simulink model "MASs"  (R2015b)
settings: Solver=ode45  SolverMode=SingleTasking  StartTime=0.0  StopTime=100000.0  RelTol=1e-3
model workspace (MAT data in the model file):
  B = 3.17
  Cb = 0.251
  Izz = 1
  L = 9.8
  d = 0.71
  m = 5540
undefined symbols (not defined in the file or in its folder): magnitude
libraries: simulink x10
(part 2 of 2)

== system MASs/usv3/USV/F model/S model ==
  u : Inport
  v : Inport  Port=2
  r : Inport  Port=3
  B : Constant  Value=B
  Cb : Constant  Value=Cb
  L : Constant  Value=L
  d : Constant  Value=d
  m : Constant  Value=m
  s-fcn : MATLAB Function  TreatAsAtomicUnit=on
  Xs : Outport
  Ys : Outport  Port=2
  Ns : Outport  Port=3
  wires:
  s-fcn/1(Xs) -> Xs/1
  s-fcn/2(Ys) -> Ys/1
  s-fcn/3(Ns) -> Ns/1
  B/1 -> s-fcn/1(B)
  d/1 -> s-fcn/2(d)
  L/1 -> s-fcn/3(L)
  u/1 -> s-fcn/6(u)
  v/1 -> s-fcn/7(v)
  r/1 -> s-fcn/8(r)
  Cb/1 -> s-fcn/4(Cb)
  m/1 -> s-fcn/5(m)

== system MASs/usv3/USV/F model/W model ==
  n : Constant  Value=0
  n1 : Constant  Value=0
  n2 : Constant  Value=0
  Xw : Outport
  Yw : Outport  Port=2
  Nw : Outport  Port=3
  wires:
  n/1 -> Xw/1
  n2/1 -> Yw/1
  n1/1 -> Nw/1

== system MASs/usv3/USV/motion model/r-sub ==
  N : Inport
  Izz : Inport  Port=2
  Jzz : Inport  Port=3
  Divide2 : Product  Inputs=*/
  Integrator2 : Integrator
  Sum4 : Sum  Inputs=|++
  r : Outport
  wires:
  Sum4/1 -> Divide2/2
  Divide2/1 -> Integrator2/1  "r'"
  Integrator2/1 -> r/1  "r"
  N/1 -> Divide2/1
  Jzz/1 -> Sum4/2
  Izz/1 -> Sum4/1

== system MASs/usv3/USV/motion model/u-sub ==
  X : Inport
  m : Inport  Port=2
  my : Inport  Port=3
  mx : Inport  Port=4
  v : Inport  Port=5
  r : Inport  Port=6
  Add : Sum
  Divide1 : Product  Inputs=*/
  Integrator : Integrator
  Product : Product  Inputs=3
  Sum : Sum  Inputs=|++
  Sum1 : Sum  Inputs=|++
  u : Outport
  wires:
  Sum1/1 -> Divide1/2
  Divide1/1 -> Integrator/1  "u'"
  Integrator/1 -> u/1  "u"
  Sum/1 -> Product/1
  Add/1 -> Divide1/1
  my/1 -> Sum/2
  X/1 -> Add/1
  v/1 -> Product/2
  r/1 -> Product/3
  mx/1 -> Sum1/2
  m/1 -> Sum1/1, Sum/1
  Product/1 -> Add/2

== system MASs/usv3/USV/motion model/v-sub ==
  Y : Inport
  m : Inport  Port=2
  mx : Inport  Port=3
  my : Inport  Port=4
  u : Inport  Port=5
  r : Inport  Port=6
  Add2 : Sum  Inputs=+-
  Divide3 : Product  Inputs=*/
  Integrator1 : Integrator
  Product1 : Product  Inputs=3
  Sum2 : Sum  Inputs=|++
  Sum3 : Sum  Inputs=|++
  v : Outport
  wires:
  Sum3/1 -> Divide3/2
  my/1 -> Sum3/1
  r/1 -> Product1/3
  Product1/1 -> Add2/2
  m/1 -> Sum3/2, Sum2/1
  Sum2/1 -> Product1/1
  Y/1 -> Add2/1
  Add2/1 -> Divide3/1
  Divide3/1 -> Integrator1/1  "v'"
  Integrator1/1 -> v/1  "v"
  u/1 -> Product1/2
  mx/1 -> Sum2/2

== system MASs/usv4/USV/F model/P model ==
  n : Inport
  δ : Inport  Port=2
  u : Inport  Port=3
  v : Inport  Port=4
  p-fcn : MATLAB Function  TreatAsAtomicUnit=on
  Xp : Outport
  Yp : Outport  Port=2
  Np : Outport  Port=3
  wires:
  p-fcn/3(Np) -> Np/1
  p-fcn/2(Yp) -> Yp/1
  p-fcn/1(Xp) -> Xp/1
  n/1 -> p-fcn/1(n)
  δ/1 -> p-fcn/2(sita)
  u/1 -> p-fcn/3(u)
  v/1 -> p-fcn/4(v)

== system MASs/usv4/USV/F model/S model ==
  u : Inport
  v : Inport  Port=2
  r : Inport  Port=3
  B : Constant  Value=B
  Cb : Constant  Value=Cb
  L : Constant  Value=L
  d : Constant  Value=d
  m : Constant  Value=m
  s-fcn : MATLAB Function  TreatAsAtomicUnit=on
  Xs : Outport
  Ys : Outport  Port=2
  Ns : Outport  Port=3
  wires:
  s-fcn/1(Xs) -> Xs/1
  s-fcn/2(Ys) -> Ys/1
  s-fcn/3(Ns) -> Ns/1
  B/1 -> s-fcn/1(B)
  d/1 -> s-fcn/2(d)
  L/1 -> s-fcn/3(L)
  u/1 -> s-fcn/6(u)
  v/1 -> s-fcn/7(v)
  r/1 -> s-fcn/8(r)
  Cb/1 -> s-fcn/4(Cb)
  m/1 -> s-fcn/5(m)

== system MASs/usv4/USV/F model/W model ==
  n : Constant  Value=0
  n1 : Constant  Value=0
  n2 : Constant  Value=0
  Xw : Outport
  Yw : Outport  Port=2
  Nw : Outport  Port=3
  wires:
  n/1 -> Xw/1
  n2/1 -> Yw/1
  n1/1 -> Nw/1

== system MASs/usv4/USV/motion model/r-sub ==
  N : Inport
  Izz : Inport  Port=2
  Jzz : Inport  Port=3
  Divide2 : Product  Inputs=*/
  Integrator2 : Integrator
  Sum4 : Sum  Inputs=|++
  r : Outport
  wires:
  Sum4/1 -> Divide2/2
  Divide2/1 -> Integrator2/1  "r'"
  Integrator2/1 -> r/1  "r"
  N/1 -> Divide2/1
  Jzz/1 -> Sum4/2
  Izz/1 -> Sum4/1

== system MASs/usv4/USV/motion model/u-sub ==
  X : Inport
  m : Inport  Port=2
  my : Inport  Port=3
  mx : Inport  Port=4
  v : Inport  Port=5
  r : Inport  Port=6
  Add : Sum
  Divide1 : Product  Inputs=*/
  Integrator : Integrator
  Product : Product  Inputs=3
  Sum : Sum  Inputs=|++
  Sum1 : Sum  Inputs=|++
  u : Outport
  wires:
  Sum1/1 -> Divide1/2
  Divide1/1 -> Integrator/1  "u'"
  Integrator/1 -> u/1  "u"
  Sum/1 -> Product/1
  Add/1 -> Divide1/1
  my/1 -> Sum/2
  X/1 -> Add/1
  v/1 -> Product/2
  r/1 -> Product/3
  mx/1 -> Sum1/2
  m/1 -> Sum1/1, Sum/1
  Product/1 -> Add/2

== system MASs/usv4/USV/motion model/v-sub ==
  Y : Inport
  m : Inport  Port=2
  mx : Inport  Port=3
  my : Inport  Port=4
  u : Inport  Port=5
  r : Inport  Port=6
  Add2 : Sum  Inputs=+-
  Divide3 : Product  Inputs=*/
  Integrator1 : Integrator
  Product1 : Product  Inputs=3
  Sum2 : Sum  Inputs=|++
  Sum3 : Sum  Inputs=|++
  v : Outport
  wires:
  Sum3/1 -> Divide3/2
  my/1 -> Sum3/1
  r/1 -> Product1/3
  Product1/1 -> Add2/2
  m/1 -> Sum3/2, Sum2/1
  Sum2/1 -> Product1/1
  Y/1 -> Add2/1
  Add2/1 -> Divide3/1
  Divide3/1 -> Integrator1/1  "v'"
  Integrator1/1 -> v/1  "v"
  u/1 -> Product1/2
  mx/1 -> Sum2/2

== system MASs/usv5/USV/F model/P model ==
  n : Inport
  δ : Inport  Port=2
  u : Inport  Port=3
  v : Inport  Port=4
  p-fcn : MATLAB Function  TreatAsAtomicUnit=on
  Xp : Outport
  Yp : Outport  Port=2
  Np : Outport  Port=3
  wires:
  p-fcn/3(Np) -> Np/1
  p-fcn/2(Yp) -> Yp/1
  p-fcn/1(Xp) -> Xp/1
  n/1 -> p-fcn/1(n)
  δ/1 -> p-fcn/2(sita)
  u/1 -> p-fcn/3(u)
  v/1 -> p-fcn/4(v)

== system MASs/usv5/USV/F model/S model ==
  u : Inport
  v : Inport  Port=2
  r : Inport  Port=3
  B : Constant  Value=B
  Cb : Constant  Value=Cb
  L : Constant  Value=L
  d : Constant  Value=d
  m : Constant  Value=m
  s-fcn : MATLAB Function  TreatAsAtomicUnit=on
  Xs : Outport
  Ys : Outport  Port=2
  Ns : Outport  Port=3
  wires:
  s-fcn/1(Xs) -> Xs/1
  s-fcn/2(Ys) -> Ys/1
  s-fcn/3(Ns) -> Ns/1
  B/1 -> s-fcn/1(B)
  d/1 -> s-fcn/2(d)
  L/1 -> s-fcn/3(L)
  u/1 -> s-fcn/6(u)
  v/1 -> s-fcn/7(v)
  r/1 -> s-fcn/8(r)
  Cb/1 -> s-fcn/4(Cb)
  m/1 -> s-fcn/5(m)

== system MASs/usv5/USV/F model/W model ==
  n : Constant  Value=0
  n1 : Constant  Value=0
  n2 : Constant  Value=0
  Xw : Outport
  Yw : Outport  Port=2
  Nw : Outport  Port=3
  wires:
  n/1 -> Xw/1
  n2/1 -> Yw/1
  n1/1 -> Nw/1

== system MASs/usv5/USV/motion model/r-sub ==
  N : Inport
  Izz : Inport  Port=2
  Jzz : Inport  Port=3
  Divide2 : Product  Inputs=*/
  Integrator2 : Integrator
  Sum4 : Sum  Inputs=|++
  r : Outport
  wires:
  Sum4/1 -> Divide2/2
  Divide2/1 -> Integrator2/1  "r'"
  Integrator2/1 -> r/1  "r"
  N/1 -> Divide2/1
  Jzz/1 -> Sum4/2
  Izz/1 -> Sum4/1

== system MASs/usv5/USV/motion model/u-sub ==
  X : Inport
  m : Inport  Port=2
  my : Inport  Port=3
  mx : Inport  Port=4
  v : Inport  Port=5
  r : Inport  Port=6
  Add : Sum
  Divide1 : Product  Inputs=*/
  Integrator : Integrator
  Product : Product  Inputs=3
  Sum : Sum  Inputs=|++
  Sum1 : Sum  Inputs=|++
  u : Outport
  wires:
  Sum1/1 -> Divide1/2
  Divide1/1 -> Integrator/1  "u'"
  Integrator/1 -> u/1  "u"
  Sum/1 -> Product/1
  Add/1 -> Divide1/1
  my/1 -> Sum/2
  X/1 -> Add/1
  v/1 -> Product/2
  r/1 -> Product/3
  mx/1 -> Sum1/2
  m/1 -> Sum1/1, Sum/1
  Product/1 -> Add/2

== system MASs/usv5/USV/motion model/v-sub ==
  Y : Inport
  m : Inport  Port=2
  mx : Inport  Port=3
  my : Inport  Port=4
  u : Inport  Port=5
  r : Inport  Port=6
  Add2 : Sum  Inputs=+-
  Divide3 : Product  Inputs=*/
  Integrator1 : Integrator
  Product1 : Product  Inputs=3
  Sum2 : Sum  Inputs=|++
  Sum3 : Sum  Inputs=|++
  v : Outport
  wires:
  Sum3/1 -> Divide3/2
  my/1 -> Sum3/1
  r/1 -> Product1/3
  Product1/1 -> Add2/2
  m/1 -> Sum3/2, Sum2/1
  Sum2/1 -> Product1/1
  Y/1 -> Add2/1
  Add2/1 -> Divide3/1
  Divide3/1 -> Integrator1/1  "v'"
  Integrator1/1 -> v/1  "v"
  u/1 -> Product1/2
  mx/1 -> Sum2/2

== matlab function MASs/usv1/USV/F model/P model/p-fcn ==
  data: n input; Xp output; sita input; Yp output; Np output; u input; v input
function [Xp, Yp, Np]= fcn(n, sita, u, v)
%#codegen
Q = 1000;  %水密度
A = 0.95;         %动量影响因子
beita = A*A;      %进口动能利用系数
C = 10;            %功率特性系数，单位千瓦
g = 9.8;          %重力加速度
np = 0.8;         %推进泵效率
Aj = pi*(0.25/2)^2;    %喷口处面积
Ain = 1.6*0.52;   %入口处管道面积
Aw = pi*0.5^2;    %弯道处管道面积
Ein = 0.01;       %进口损失系数
En = 0.02;        %水力损失系数
E0 = 0.01;        %弯道损失系数
h = 0.6;          %喷口高度损失

Xt = 3;    %推力作用点在舰体坐标系下的坐标

sita = sita*pi/180;
Vs = (u^2+v^2)^(1/2); %船的航速

p = Q*Aj*(1/2+Ein/2*(Aj/Ain)^2+En/2+E0/2*(Aj/Aw)^2);
q = Q*g*Aj*(h-beita*Vs^2/(2*g));
r = -C*(n/1000)^3*np;

%p = g*(h-beita*Vs^2/(2*g))/(1/2+Ein/2*(Aj/Ain)^2+En/2+E0/2*(Aj/Aw)^2);
%q = -C*(n/1000)^3*np/(Q*Aj*(1/2+Ein/2*(Aj/Ain)^2+En/2+E0/2*(Aj/Aw)^2));
%Vj = (-q/2-((q/2)^2+(p/3)^3)^(1/2))^(1/3) + (-q/2+((q/2)^2+(p/3)^3)^(1/2))^(1/3);
V = roots([p 0 q r]);
Vj = 0;

for i=1:size(V,1)
    if imag(V(i)) < 10^(-10)
        Vj = real(V(i));
    end
end
Xp = Q*Aj*Vj*(Vj-A*Vs)*cos(sita);
Yp = Q*Aj*Vj*(Vj-A*Vs)*sin(sita);
Np = Yp*Xt;

== matlab function MASs/usv1/USV/F model/S model/s-fcn ==
  data: B input; Xs output; d input; L input; Cb input; m input; Ys output; Ns output; u input; v input; r input
function [Xs, Ys, Ns]= fcn(B, d, L, Cb, m, u, v, r)
%#codegen
P = 1000;
K = 2*d/L;
dA = 0.67;
df = 0.72;
d1 = dA-df;
d2 = (dA+df)/2;
t = d1/d2; 
U = (u^2+v^2)^(1/2);
deta = m/1025;
S = (3.14^(deta/3)+0.5*L)^(1/3);
vv = 1.07854*10^(-6);
Re = L*U/vv;
Cf = 0.075/(log10(Re)-2)^2;
Ks = 150*10^(-6);
deCf = (105*(Ks/L)^(1/3)-0.64)*10^(-3);

Xu = 0.5*P*S*u^2*(Cf+deCf);
Yv = -1/2*P*L*d*U*((0.5*pi*K+1.4*Cb*B/L)*(1+0.67*t/d));
Yr = 1/2*P*L*L*d*U*(0.25*pi*K*(1+0.8*t/d));
Nv = -1/2*P*L*L*d*U*(K-0.27*(0.5*pi+1.4*Cb*B/L)*t/d);
Nr = 1/2*P*L^3*d*U*(-(0.54*K-K^2)*(1+0.3*t/d));

Xs = Xu;
Ys = Yv*v + Yr*r;
Ns = Nv*v + Nr*r;

== matlab function MASs/usv1/USV/M model/Jzz_Fcn ==
  data: m input; Jzz output; B input; L input; Cb input
function Jzz = fcn(m, B, L, Cb)
%#codegen
temp = 33 - 76.85*Cb*(1-0.784*Cb) + 3.43*(1-0.63*Cb)*L/B;
Jzz = temp*m*L*L/100;

== matlab function MASs/usv1/USV/M model/mx_Fcn ==
  data: m input; mx output; B input; L input; d input; Cb input
function mx = fcn(m, B, L, d, Cb)
%#codegen
temp = 0.398 + 11.97*Cb*(1+3.73*d/B) - 2.89*Cb*(1+1.13*d/B) + 0.175*Cb*(L/B)^2*(1+0.541*d/B) - 1.107*L*d/(B*B);
mx = temp*m/100;

== matlab function MASs/usv1/USV/M model/my_Fcn ==
  data: m input; my output; B input; L input; d input; Cb input
function my = fcn(m, B, L, d, Cb)
%#codegen
temp = 0.882 - 0.54*Cb*(1-1.6*d/B) - 0.156*Cb*(1-0.673*Cb)*d/B + 0.826*d*L/(B*B)*(1-0.678*d/B) - 0.638*Cb*d*L/(B*B)*(1-0.619*d/B);
my = temp*m;

== matlab function MASs/usv1/USV/motion model/dx ==
  data: u input; dx output; v input; fai input
function dx = fcn(u, v, fai)
%#codegen
dx = u*cos(fai) - v*sin(fai);

== matlab function MASs/usv1/USV/motion model/dy ==
  data: u input; dy output; v input; fai input
function dy = fcn(u, v, fai)
%#codegen
dy = u*sin(fai) + v*cos(fai);

== matlab function MASs/usv2/USV/F model/P model/p-fcn ==
  data: n input; Xp output; sita input; Yp output; Np output; u input; v input
function [Xp, Yp, Np]= fcn(n, sita, u, v)
%#codegen
Q = 1000;  %水密度
A = 0.95;         %动量影响因子
beita = A*A;      %进口动能利用系数
C = 10;            %功率特性系数，单位千瓦
g = 9.8;          %重力加速度
np = 0.8;         %推进泵效率
Aj = pi*(0.25/2)^2;    %喷口处面积
Ain = 1.6*0.52;   %入口处管道面积
Aw = pi*0.5^2;    %弯道处管道面积
Ein = 0.01;       %进口损失系数
En = 0.02;        %水力损失系数
E0 = 0.01;        %弯道损失系数
h = 0.6;          %喷口高度损失

Xt = 3;    %推力作用点在舰体坐标系下的坐标

sita = sita*pi/180;
Vs = (u^2+v^2)^(1/2); %船的航速

p = Q*Aj*(1/2+Ein/2*(Aj/Ain)^2+En/2+E0/2*(Aj/Aw)^2);
q = Q*g*Aj*(h-beita*Vs^2/(2*g));
r = -C*(n/1000)^3*np;

%p = g*(h-beita*Vs^2/(2*g))/(1/2+Ein/2*(Aj/Ain)^2+En/2+E0/2*(Aj/Aw)^2);
%q = -C*(n/1000)^3*np/(Q*Aj*(1/2+Ein/2*(Aj/Ain)^2+En/2+E0/2*(Aj/Aw)^2));
%Vj = (-q/2-((q/2)^2+(p/3)^3)^(1/2))^(1/3) + (-q/2+((q/2)^2+(p/3)^3)^(1/2))^(1/3);
V = roots([p 0 q r]);
Vj = 0;

for i=1:size(V,1)
    if imag(V(i)) < 10^(-10)
        Vj = real(V(i));
    end
end
Xp = Q*Aj*Vj*(Vj-A*Vs)*cos(sita);
Yp = Q*Aj*Vj*(Vj-A*Vs)*sin(sita);
Np = Yp*Xt;

== matlab function MASs/usv2/USV/F model/S model/s-fcn ==
  data: B input; Xs output; d input; L input; Cb input; m input; Ys output; Ns output; u input; v input; r input
function [Xs, Ys, Ns]= fcn(B, d, L, Cb, m, u, v, r)
%#codegen
P = 1000;
K = 2*d/L;
dA = 0.67;
df = 0.72;
d1 = dA-df;
d2 = (dA+df)/2;
t = d1/d2; 
U = (u^2+v^2)^(1/2);
deta = m/1025;
S = (3.14^(deta/3)+0.5*L)^(1/3);
vv = 1.07854*10^(-6);
Re = L*U/vv;
Cf = 0.075/(log10(Re)-2)^2;
Ks = 150*10^(-6);
deCf = (105*(Ks/L)^(1/3)-0.64)*10^(-3);

Xu = 0.5*P*S*u^2*(Cf+deCf);
Yv = -1/2*P*L*d*U*((0.5*pi*K+1.4*Cb*B/L)*(1+0.67*t/d));
Yr = 1/2*P*L*L*d*U*(0.25*pi*K*(1+0.8*t/d));
Nv = -1/2*P*L*L*d*U*(K-0.27*(0.5*pi+1.4*Cb*B/L)*t/d);
Nr = 1/2*P*L^3*d*U*(-(0.54*K-K^2)*(1+0.3*t/d));

Xs = Xu;
Ys = Yv*v + Yr*r;
Ns = Nv*v + Nr*r;

== matlab function MASs/usv2/USV/M model/Jzz_Fcn ==
  data: m input; Jzz output; B input; L input; Cb input
function Jzz = fcn(m, B, L, Cb)
%#codegen
temp = 33 - 76.85*Cb*(1-0.784*Cb) + 3.43*(1-0.63*Cb)*L/B;
Jzz = temp*m*L*L/100;

== matlab function MASs/usv2/USV/M model/mx_Fcn ==
  data: m input; mx output; B input; L input; d input; Cb input
function mx = fcn(m, B, L, d, Cb)
%#codegen
temp = 0.398 + 11.97*Cb*(1+3.73*d/B) - 2.89*Cb*(1+1.13*d/B) + 0.175*Cb*(L/B)^2*(1+0.541*d/B) - 1.107*L*d/(B*B);
mx = temp*m/100;

== matlab function MASs/usv2/USV/M model/my_Fcn ==
  data: m input; my output; B input; L input; d input; Cb input
function my = fcn(m, B, L, d, Cb)
%#codegen
temp = 0.882 - 0.54*Cb*(1-1.6*d/B) - 0.156*Cb*(1-0.673*Cb)*d/B + 0.826*d*L/(B*B)*(1-0.678*d/B) - 0.638*Cb*d*L/(B*B)*(1-0.619*d/B);
my = temp*m;

== matlab function MASs/usv2/USV/motion model/dx ==
  data: u input; dx output; v input; fai input
function dx = fcn(u, v, fai)
%#codegen
dx = u*cos(fai) - v*sin(fai);

== matlab function MASs/usv2/USV/motion model/dy ==
  data: u input; dy output; v input; fai input
function dy = fcn(u, v, fai)
%#codegen
dy = u*sin(fai) + v*cos(fai);

== matlab function MASs/usv4/USV/F model/P model/p-fcn ==
  data: n input; Xp output; sita input; Yp output; Np output; u input; v input
function [Xp, Yp, Np]= fcn(n, sita, u, v)
%#codegen
Q = 1000;  %水密度
A = 0.95;         %动量影响因子
beita = A*A;      %进口动能利用系数
C = 10;            %功率特性系数，单位千瓦
g = 9.8;          %重力加速度
np = 0.8;         %推进泵效率
Aj = pi*(0.25/2)^2;    %喷口处面积
Ain = 1.6*0.52;   %入口处管道面积
Aw = pi*0.5^2;    %弯道处管道面积
Ein = 0.01;       %进口损失系数
En = 0.02;        %水力损失系数
E0 = 0.01;        %弯道损失系数
h = 0.6;          %喷口高度损失

Xt = 3;    %推力作用点在舰体坐标系下的坐标

sita = sita*pi/180;
Vs = (u^2+v^2)^(1/2); %船的航速

p = Q*Aj*(1/2+Ein/2*(Aj/Ain)^2+En/2+E0/2*(Aj/Aw)^2);
q = Q*g*Aj*(h-beita*Vs^2/(2*g));
r = -C*(n/1000)^3*np;

%p = g*(h-beita*Vs^2/(2*g))/(1/2+Ein/2*(Aj/Ain)^2+En/2+E0/2*(Aj/Aw)^2);
%q = -C*(n/1000)^3*np/(Q*Aj*(1/2+Ein/2*(Aj/Ain)^2+En/2+E0/2*(Aj/Aw)^2));
%Vj = (-q/2-((q/2)^2+(p/3)^3)^(1/2))^(1/3) + (-q/2+((q/2)^2+(p/3)^3)^(1/2))^(1/3);
V = roots([p 0 q r]);
Vj = 0;

for i=1:size(V,1)
    if imag(V(i)) < 10^(-10)
        Vj = real(V(i));
    end
end
Xp = Q*Aj*Vj*(Vj-A*Vs)*cos(sita);
Yp = Q*Aj*Vj*(Vj-A*Vs)*sin(sita);
Np = Yp*Xt;

== matlab function MASs/usv4/USV/F model/S model/s-fcn ==
  data: B input; Xs output; d input; L input; Cb input; m input; Ys output; Ns output; u input; v input; r input
function [Xs, Ys, Ns]= fcn(B, d, L, Cb, m, u, v, r)
%#codegen
P = 1000;
K = 2*d/L;
dA = 0.67;
df = 0.72;
d1 = dA-df;
d2 = (dA+df)/2;
t = d1/d2; 
U = (u^2+v^2)^(1/2);
deta = m/1025;
S = (3.14^(deta/3)+0.5*L)^(1/3);
vv = 1.07854*10^(-6);
Re = L*U/vv;
Cf = 0.075/(log10(Re)-2)^2;
Ks = 150*10^(-6);
deCf = (105*(Ks/L)^(1/3)-0.64)*10^(-3);

Xu = 0.5*P*S*u^2*(Cf+deCf);
Yv = -1/2*P*L*d*U*((0.5*pi*K+1.4*Cb*B/L)*(1+0.67*t/d));
Yr = 1/2*P*L*L*d*U*(0.25*pi*K*(1+0.8*t/d));
Nv = -1/2*P*L*L*d*U*(K-0.27*(0.5*pi+1.4*Cb*B/L)*t/d);
Nr = 1/2*P*L^3*d*U*(-(0.54*K-K^2)*(1+0.3*t/d));

Xs = Xu;
Ys = Yv*v + Yr*r;
Ns = Nv*v + Nr*r;

== matlab function MASs/usv4/USV/M model/Jzz_Fcn ==
  data: m input; Jzz output; B input; L input; Cb input
function Jzz = fcn(m, B, L, Cb)
%#codegen
temp = 33 - 76.85*Cb*(1-0.784*Cb) + 3.43*(1-0.63*Cb)*L/B;
Jzz = temp*m*L*L/100;

== matlab function MASs/usv4/USV/M model/mx_Fcn ==
  data: m input; mx output; B input; L input; d input; Cb input
function mx = fcn(m, B, L, d, Cb)
%#codegen
temp = 0.398 + 11.97*Cb*(1+3.73*d/B) - 2.89*Cb*(1+1.13*d/B) + 0.175*Cb*(L/B)^2*(1+0.541*d/B) - 1.107*L*d/(B*B);
mx = temp*m/100;

== matlab function MASs/usv4/USV/M model/my_Fcn ==
  data: m input; my output; B input; L input; d input; Cb input
function my = fcn(m, B, L, d, Cb)
%#codegen
temp = 0.882 - 0.54*Cb*(1-1.6*d/B) - 0.156*Cb*(1-0.673*Cb)*d/B + 0.826*d*L/(B*B)*(1-0.678*d/B) - 0.638*Cb*d*L/(B*B)*(1-0.619*d/B);
my = temp*m;

== matlab function MASs/usv4/USV/motion model/dx ==
  data: u input; dx output; v input; fai input
function dx = fcn(u, v, fai)
%#codegen
dx = u*cos(fai) - v*sin(fai);

== matlab function MASs/usv4/USV/motion model/dy ==
  data: u input; dy output; v input; fai input
function dy = fcn(u, v, fai)
%#codegen
dy = u*sin(fai) + v*cos(fai);

== matlab function MASs/usv3/USV/F model/P model/p-fcn ==
  data: n input; Xp output; sita input; Yp output; Np output; u input; v input
function [Xp, Yp, Np]= fcn(n, sita, u, v)
%#codegen
Q = 1000;  %水密度
A = 0.95;         %动量影响因子
beita = A*A;      %进口动能利用系数
C = 10;            %功率特性系数，单位千瓦
g = 9.8;          %重力加速度
np = 0.8;         %推进泵效率
Aj = pi*(0.25/2)^2;    %喷口处面积
Ain = 1.6*0.52;   %入口处管道面积
Aw = pi*0.5^2;    %弯道处管道面积
Ein = 0.01;       %进口损失系数
En = 0.02;        %水力损失系数
E0 = 0.01;        %弯道损失系数
h = 0.6;          %喷口高度损失

Xt = 3;    %推力作用点在舰体坐标系下的坐标

sita = sita*pi/180;
Vs = (u^2+v^2)^(1/2); %船的航速

p = Q*Aj*(1/2+Ein/2*(Aj/Ain)^2+En/2+E0/2*(Aj/Aw)^2);
q = Q*g*Aj*(h-beita*Vs^2/(2*g));
r = -C*(n/1000)^3*np;

%p = g*(h-beita*Vs^2/(2*g))/(1/2+Ein/2*(Aj/Ain)^2+En/2+E0/2*(Aj/Aw)^2);
%q = -C*(n/1000)^3*np/(Q*Aj*(1/2+Ein/2*(Aj/Ain)^2+En/2+E0/2*(Aj/Aw)^2));
%Vj = (-q/2-((q/2)^2+(p/3)^3)^(1/2))^(1/3) + (-q/2+((q/2)^2+(p/3)^3)^(1/2))^(1/3);
V = roots([p 0 q r]);
Vj = 0;

for i=1:size(V,1)
    if imag(V(i)) < 10^(-10)
        Vj = real(V(i));
    end
end
Xp = Q*Aj*Vj*(Vj-A*Vs)*cos(sita);
Yp = Q*Aj*Vj*(Vj-A*Vs)*sin(sita);
Np = Yp*Xt;

== matlab function MASs/usv3/USV/F model/S model/s-fcn ==
  data: B input; Xs output; d input; L input; Cb input; m input; Ys output; Ns output; u input; v input; r input
function [Xs, Ys, Ns]= fcn(B, d, L, Cb, m, u, v, r)
%#codegen
P = 1000;
K = 2*d/L;
dA = 0.67;
df = 0.72;
d1 = dA-df;
d2 = (dA+df)/2;
t = d1/d2; 
U = (u^2+v^2)^(1/2);
deta = m/1025;
S = (3.14^(deta/3)+0.5*L)^(1/3);
vv = 1.07854*10^(-6);
Re = L*U/vv;
Cf = 0.075/(log10(Re)-2)^2;
Ks = 150*10^(-6);
deCf = (105*(Ks/L)^(1/3)-0.64)*10^(-3);

Xu = 0.5*P*S*u^2*(Cf+deCf);
Yv = -1/2*P*L*d*U*((0.5*pi*K+1.4*Cb*B/L)*(1+0.67*t/d));
Yr = 1/2*P*L*L*d*U*(0.25*pi*K*(1+0.8*t/d));
Nv = -1/2*P*L*L*d*U*(K-0.27*(0.5*pi+1.4*Cb*B/L)*t/d);
Nr = 1/2*P*L^3*d*U*(-(0.54*K-K^2)*(1+0.3*t/d));

Xs = Xu;
Ys = Yv*v + Yr*r;
Ns = Nv*v + Nr*r;

== matlab function MASs/usv3/USV/M model/Jzz_Fcn ==
  data: m input; Jzz output; B input; L input; Cb input
function Jzz = fcn(m, B, L, Cb)
%#codegen
temp = 33 - 76.85*Cb*(1-0.784*Cb) + 3.43*(1-0.63*Cb)*L/B;
Jzz = temp*m*L*L/100;

== matlab function MASs/usv3/USV/M model/mx_Fcn ==
  data: m input; mx output; B input; L input; d input; Cb input
function mx = fcn(m, B, L, d, Cb)
%#codegen
temp = 0.398 + 11.97*Cb*(1+3.73*d/B) - 2.89*Cb*(1+1.13*d/B) + 0.175*Cb*(L/B)^2*(1+0.541*d/B) - 1.107*L*d/(B*B);
mx = temp*m/100;

== matlab function MASs/usv3/USV/M model/my_Fcn ==
  data: m input; my output; B input; L input; d input; Cb input
function my = fcn(m, B, L, d, Cb)
%#codegen
temp = 0.882 - 0.54*Cb*(1-1.6*d/B) - 0.156*Cb*(1-0.673*Cb)*d/B + 0.826*d*L/(B*B)*(1-0.678*d/B) - 0.638*Cb*d*L/(B*B)*(1-0.619*d/B);
my = temp*m;

== matlab function MASs/usv3/USV/motion model/dx ==
  data: u input; dx output; v input; fai input
function dx = fcn(u, v, fai)
%#codegen
dx = u*cos(fai) - v*sin(fai);

== matlab function MASs/usv3/USV/motion model/dy ==
  data: u input; dy output; v input; fai input
function dy = fcn(u, v, fai)
%#codegen
dy = u*sin(fai) + v*cos(fai);

== matlab function MASs/usv5/USV/F model/P model/p-fcn ==
  data: n input; Xp output; sita input; Yp output; Np output; u input; v input
function [Xp, Yp, Np]= fcn(n, sita, u, v)
%#codegen
Q = 1000;  %水密度
A = 0.95;         %动量影响因子
beita = A*A;      %进口动能利用系数
C = 10;            %功率特性系数，单位千瓦
g = 9.8;          %重力加速度
np = 0.8;         %推进泵效率
Aj = pi*(0.25/2)^2;    %喷口处面积
Ain = 1.6*0.52;   %入口处管道面积
Aw = pi*0.5^2;    %弯道处管道面积
Ein = 0.01;       %进口损失系数
En = 0.02;        %水力损失系数
E0 = 0.01;        %弯道损失系数
h = 0.6;          %喷口高度损失

Xt = 3;    %推力作用点在舰体坐标系下的坐标

sita = sita*pi/180;
Vs = (u^2+v^2)^(1/2); %船的航速

p = Q*Aj*(1/2+Ein/2*(Aj/Ain)^2+En/2+E0/2*(Aj/Aw)^2);
q = Q*g*Aj*(h-beita*Vs^2/(2*g));
r = -C*(n/1000)^3*np;

%p = g*(h-beita*Vs^2/(2*g))/(1/2+Ein/2*(Aj/Ain)^2+En/2+E0/2*(Aj/Aw)^2);
%q = -C*(n/1000)^3*np/(Q*Aj*(1/2+Ein/2*(Aj/Ain)^2+En/2+E0/2*(Aj/Aw)^2));
%Vj = (-q/2-((q/2)^2+(p/3)^3)^(1/2))^(1/3) + (-q/2+((q/2)^2+(p/3)^3)^(1/2))^(1/3);
V = roots([p 0 q r]);
Vj = 0;

for i=1:size(V,1)
    if imag(V(i)) < 10^(-10)
        Vj = real(V(i));
    end
end
Xp = Q*Aj*Vj*(Vj-A*Vs)*cos(sita);
Yp = Q*Aj*Vj*(Vj-A*Vs)*sin(sita);
Np = Yp*Xt;

== matlab function MASs/usv5/USV/F model/S model/s-fcn ==
  data: B input; Xs output; d input; L input; Cb input; m input; Ys output; Ns output; u input; v input; r input
function [Xs, Ys, Ns]= fcn(B, d, L, Cb, m, u, v, r)
%#codegen
P = 1000;
K = 2*d/L;
dA = 0.67;
df = 0.72;
d1 = dA-df;
d2 = (dA+df)/2;
t = d1/d2; 
U = (u^2+v^2)^(1/2);
deta = m/1025;
S = (3.14^(deta/3)+0.5*L)^(1/3);
vv = 1.07854*10^(-6);
Re = L*U/vv;
Cf = 0.075/(log10(Re)-2)^2;
Ks = 150*10^(-6);
deCf = (105*(Ks/L)^(1/3)-0.64)*10^(-3);

Xu = 0.5*P*S*u^2*(Cf+deCf);
Yv = -1/2*P*L*d*U*((0.5*pi*K+1.4*Cb*B/L)*(1+0.67*t/d));
Yr = 1/2*P*L*L*d*U*(0.25*pi*K*(1+0.8*t/d));
Nv = -1/2*P*L*L*d*U*(K-0.27*(0.5*pi+1.4*Cb*B/L)*t/d);
Nr = 1/2*P*L^3*d*U*(-(0.54*K-K^2)*(1+0.3*t/d));

Xs = Xu;
Ys = Yv*v + Yr*r;
Ns = Nv*v + Nr*r;

== matlab function MASs/usv5/USV/M model/Jzz_Fcn ==
  data: m input; Jzz output; B input; L input; Cb input
function Jzz = fcn(m, B, L, Cb)
%#codegen
temp = 33 - 76.85*Cb*(1-0.784*Cb) + 3.43*(1-0.63*Cb)*L/B;
Jzz = temp*m*L*L/100;

== matlab function MASs/usv5/USV/M model/mx_Fcn ==
  data: m input; mx output; B input; L input; d input; Cb input
function mx = fcn(m, B, L, d, Cb)
%#codegen
temp = 0.398 + 11.97*Cb*(1+3.73*d/B) - 2.89*Cb*(1+1.13*d/B) + 0.175*Cb*(L/B)^2*(1+0.541*d/B) - 1.107*L*d/(B*B);
mx = temp*m/100;

== matlab function MASs/usv5/USV/M model/my_Fcn ==
  data: m input; my output; B input; L input; d input; Cb input
function my = fcn(m, B, L, d, Cb)
%#codegen
temp = 0.882 - 0.54*Cb*(1-1.6*d/B) - 0.156*Cb*(1-0.673*Cb)*d/B + 0.826*d*L/(B*B)*(1-0.678*d/B) - 0.638*Cb*d*L/(B*B)*(1-0.619*d/B);
my = temp*m;

== matlab function MASs/usv5/USV/motion model/dx ==
  data: u input; dx output; v input; fai input
function dx = fcn(u, v, fai)
%#codegen
dx = u*cos(fai) - v*sin(fai);

== matlab function MASs/usv5/USV/motion model/dy ==
  data: u input; dy output; v input; fai input
function dy = fcn(u, v, fai)
%#codegen
dy = u*sin(fai) + v*cos(fai);
